simulink model "cooling_model"  (R2022a)
settings: Solver=VariableStepAuto  StartTime=4192  StopTime=20000  RelTol=1e-3
values from neighbouring files (symbols this model uses):
  area_air_fan = (fan_qty*pi.*fan_dia^2)./4'    [Cooling_Script.m]
  area_fins = n_fins * (h_fin-delta_fin) * w_radiator * 2    [Cooling_Script.m]
  area_fins_inverter = n_fins_inverter * (h_fin_inverter-delta_fin_inverter) * w_radiator_inverter * 2    [Cooling_Script.m]
  area_fins_motor = n_fins_motor * (h_fin_motor-delta_fin_motor) * w_radiator_motor * 2    [Cooling_Script.m]
  area_primary = 2 * L_tube * w_radiator * (n_fin_rows) - 2 * delta_fin * w_radiator * n_fins + 2 * h_fin * w_radiator * n_fin_rows + 2 * h_tube * n_tubes * L_tube    [Cooling_Script.m]
  area_primary_inverter = 2 * L_tube_inverter * w_radiator_inverter * (n_fin_rows_inverter) - 2 * delta_fin_inverter * w_radiator_inverter * n_fins_inverter + 2 * h_fin_inverter * w_radiator_inverter * n_fin_rows_inverter + 2 * h_tube_inverter * n_tubes_inverter * L_tube_inverter    [Cooling_Script.m]
  area_primary_motor = 2 * L_tube_motor * w_radiator_motor * (n_fin_rows_motor) - 2 * delta_fin_motor * w_radiator_motor * n_fins_motor + 2 * h_fin_motor * w_radiator_motor * n_fin_rows_motor + 2 * h_tube_motor * n_tubes_motor * L_tube_motor    [Cooling_Script.m]
  cp_air = 1004    [Cooling_Script.m]
  h_tube = 0.0015    [Cooling_Script.m]
  h_tube_inverter = 0.0015    [Cooling_Script.m]
  h_tube_motor = 0.0015    [Cooling_Script.m]
  HC_min = 10    [Cooling_Script.m]
  HC_nom = 100    [Cooling_Script.m]
  L_tube = 46*25.4./1000    [Cooling_Script.m]
  L_tube_inverter = 46*25.4./1000    [Cooling_Script.m]
  L_tube_motor = 46*25.4./1000    [Cooling_Script.m]
  n_tubes = 36    [Cooling_Script.m]
  n_tubes_inverter = 36    [Cooling_Script.m]
  n_tubes_motor = 36    [Cooling_Script.m]
  rho_air = 1.2    [Cooling_Script.m]
  vel_air_nom = 1    [Cooling_Script.m]
  w_radiator = 2.6*25.4    (= 66.04)    [Cooling_Script.m]
  w_radiator_inverter = 2.6*25.4    (= 66.04)    [Cooling_Script.m]
  w_radiator_motor = 2.6*25.4    (= 66.04)    [Cooling_Script.m]
libraries: fl_lib x65, nesl_utility x35, SimscapeFluids_lib x12, aerolibconvert2 x9
(part 2 of 2)

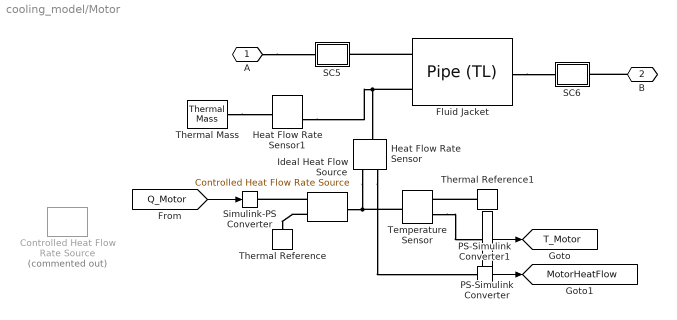
== system cooling_model/Motor ==
  Controlled Heat Flow Rate Source : fl_lib/Thermal/Thermal Sources/Controlled Heat Flow Rate Source  Commented=on
      settings: SourceProductBaseCode=PW,SS,VE
  Fluid Jacket : SimscapeFluids_lib/Thermal Liquid/Pipes & Fittings/Pipe (TL)  dynamic_compressibility=simscape.enum.onoff.off  inertia=simscape.enum.onoff.off  num_segments=1  pipe_length=0.2 m  area=pi*0.01^2 m^2  wall_spec=fluids.thermal_liquid.pipes_fittings.enum.wall_spec.rigid  Dh=0.005 m  wall_compliance=1.2e-6 m/MPa  wall_time_constant=0.01 s  elevation_spec=foundation.enum.constant_variable.constant  elevation_gain=0 m  g=9.81 m/s^2  pressure_loss_spec=fluids.thermal_liquid.pipes_fittings.enum.PressureLossSpec.Nominal  local_pressure_loss_spec=fluids.thermal_liquid.pipes_fittings.enum.LocalLossSpec.AggregateLength  length_add=0 m  loss_coefficient=0.1  roughness=1.5e-60 m  Re_friction_TLU=[ 400 1000 1.5e+3 3e+3 4e+3 6e+3 1e+4 2e+4 4e+4 6e+4 1e+5 1e+8 ]  friction_factor_TLU=[ 0.264 0.112 0.07099999999999999 0.0417 0.0387 0.0268 0.025 0.0232 0.0226 0.022 0.0214 0.0214 ]  shape_factor=1e-50  Re_lam=2e+3  Re_tur=4e+3  mdot_nominal=[ 0.1 1000 ] kg/s  p_diff_nominal=[ 0.00000001 0.000000001 ] MPa  mdot_threshold=1e-6 kg/s  heat_transfer_spec=fluids.thermal_liquid.pipes_fittings.enum.HeatTransferSpec.TabulatedNusselt  mdot_nominal_heat=[ 0.1 1 ] kg/s  T_in_nominal=[ 293.15 293.15 ] K  T_out_nominal=[ 300 300 ] K  p_in_nominal_heat=[ 0.101325 0.101325 ] MPa  T_wall_nominal=[ 303.15 303.15 ] K  a_coeff=0.023  b_Re_power=0.8  c_Pr_power=0.4  Nu_lam=3.66  Re_Colburn_TLU=[ 100 150 1000 ]  Colburn_factor_TLU=[ 0.019 0.013 0.002 ]  Re_Nu_TLU=Re_TLU  Pr_Nu_TLU=Pr_TLU  Nu_TLU=Nu_TLU  T0_vec=303.15 K  p0_vec=0.101325 MPa  mdot0=0.1 kg/s
      settings: SourceProductBaseCode=SH
  Heat Flow Rate Sensor : fl_lib/Thermal/Thermal Sensors/Heat Flow Rate Sensor
      settings: SourceProductBaseCode=PW,SS,VE
  Heat Flow Rate Sensor1 : fl_lib/Thermal/Thermal Sensors/Heat Flow Rate Sensor
      settings: SourceProductBaseCode=PW,SS,VE
  Ideal Heat Flow Source : fl_lib/Thermal/Thermal Sources/Controlled Heat Flow Rate Source
      settings: SourceProductBaseCode=PW,SS,VE
  PS-Simulink Converter : nesl_utility/PS-Simulink Converter  PhysicalDomain=network_engine_domain  SubClassName=ps_output  LeftPortType=input  RightPortType=output  PseudoPeriodic=off  Frequencies=[]  VectorFormat=1-D array  Unit=degC  AffineConversion=on
      settings: SourceProductBaseCode=SS,PW,VE
  PS-Simulink Converter1 : nesl_utility/PS-Simulink Converter  PhysicalDomain=network_engine_domain  SubClassName=ps_output  LeftPortType=input  RightPortType=output  PseudoPeriodic=off  Frequencies=[]  VectorFormat=inherit  Unit=inherit  AffineConversion=off
      settings: SourceProductBaseCode=SS,PW,VE
  SC5 : Subsystem
      mask Display: disp(get_param(gcb, 'Name'))
  SC6 : Subsystem
      mask Display: disp(get_param(gcb, 'Name'))
  Simulink-PS Converter : nesl_utility/Simulink-PS Converter  PhysicalDomain=network_engine_domain  SubClassName=ps_input  LeftPortType=input  RightPortType=output  PseudoPeriodic=off  Frequencies=[]  NoiseDistribution=none  NoiseParameters=[]  Unit=W  AffineConversion=off  FilteringAndDerivatives=provide  SimscapeFilterOrder=1  InputFilterTimeConstant=0.001  UdotUserProvided=0
      settings: SourceProductBaseCode=SS,PW,VE
  Temperature Sensor : fl_lib/Thermal/Thermal Sensors/Temperature Sensor
      settings: SourceProductBaseCode=PW,SS,VE
  Thermal Mass : fl_lib/Thermal/Thermal Elements/Thermal Mass  mass=28.5*6 kg  sp_heat=447 J/(K*kg)  T_specify=on  T_priority=High  T=273+45 K  T_nominal_specify=on  T_nominal_unit=K  T_nominal_value=273.15+45  Q_specify=off  Q_priority=None  Q=0 W  Q_nominal_specify=off  Q_nominal_unit=W  Q_nominal_value=1
      settings: SourceProductBaseCode=PW,SS,VE
  Thermal Reference : fl_lib/Thermal/Thermal Elements/Thermal Reference
      settings: SourceProductBaseCode=PW,SS,VE
  Thermal Reference1 : fl_lib/Thermal/Thermal Elements/Thermal Reference
      settings: SourceProductBaseCode=PW,SS,VE
  A : PMIOPort  Side=Left
  B : PMIOPort  Port=2  Side=Right
  tag scope: MotorHeatFlow=global, T_Motor=global
  wires:
  [Q_Motor] -> Simulink-PS Converter/1
  PS-Simulink Converter/1 -> [T_Motor]
  PS-Simulink Converter1/1 -> [MotorHeatFlow]
  connections:
  Temperature Sensor/LConn1 -- Heat Flow Rate Sensor/RConn2 -- Ideal Heat Flow Source/LConn1
  B/RConn1 -- SC6/RConn1
  Ideal Heat Flow Source/RConn2 -- Thermal Reference/LConn1
  A/RConn1 -- SC5/LConn1
  Ideal Heat Flow Source/RConn1 -- Simulink-PS Converter/RConn1
  Thermal Reference1/LConn1 -- Temperature Sensor/RConn1
  Temperature Sensor/RConn2 -- PS-Simulink Converter/LConn1
  Fluid Jacket/LConn2 -- Heat Flow Rate Sensor1/RConn2 -- Heat Flow Rate Sensor/LConn1
  Heat Flow Rate Sensor/RConn1 -- PS-Simulink Converter1/LConn1
  Fluid Jacket/LConn1 -- SC5/RConn1
  Fluid Jacket/RConn1 -- SC6/LConn1
  Thermal Mass/LConn1 -- Heat Flow Rate Sensor1/LConn1

== system cooling_model/Sensing Coolant1 ==
  Absolute Reference (TL) : fl_lib/Thermal Liquid/Elements/Absolute Reference (TL)
      settings: SourceProductBaseCode=PW,SS,VE
  PS-Simulink Converter : nesl_utility/PS-Simulink Converter  PhysicalDomain=network_engine_domain  SubClassName=ps_output  LeftPortType=input  RightPortType=output  PseudoPeriodic=off  Frequencies=[]  VectorFormat=1-D array  Unit=K  AffineConversion=on
      settings: SourceProductBaseCode=SS,PW,VE
  Pressure & Temperature Sensor (TL) : fl_lib/Thermal Liquid/Sensors/Pressure & Temperature Sensor (TL)
      settings: SourceProductBaseCode=PW,SS,VE  InternalSimscapePortConfiguration="{\"Bottom\":[],\"Left\":[{\"id\":\"A\",\"label\":\"A\",\"type\":\"foundation.thermal_liquid.thermal_liquid\"}],\"Right\":[{\"id\":\"B\",\"label\":\"B\",\"type\":\"foundation.thermal_liquid.thermal_liquid\"},{\"id\":\"P\",\"label\":\"P\",\"type\":\"output\"},{\"id\":\"T\",\"label\":\"T\",\"type\":\"output\"}],\"Top\":[]}"
  Conn1 : PMIOPort  Side=Left
  Out1 : Outport  VectorParamsAs1DForOutWhenUnconnected=off
  wires:
  PS-Simulink Converter/1 -> Out1/1
  connections:
  Pressure & Temperature Sensor (TL)/LConn1 -- Conn1/RConn1
  PS-Simulink Converter/LConn1 -- Pressure & Temperature Sensor (TL)/RConn3
  Pressure & Temperature Sensor (TL)/RConn1 -- Absolute Reference (TL)/LConn1

== system cooling_model/Sensing Coolant2 ==
  Absolute Reference (TL) : fl_lib/Thermal Liquid/Elements/Absolute Reference (TL)
      settings: SourceProductBaseCode=PW,SS,VE
  PS-Simulink Converter : nesl_utility/PS-Simulink Converter  PhysicalDomain=network_engine_domain  SubClassName=ps_output  LeftPortType=input  RightPortType=output  PseudoPeriodic=off  Frequencies=[]  VectorFormat=1-D array  Unit=K  AffineConversion=on
      settings: SourceProductBaseCode=SS,PW,VE
  Pressure & Temperature Sensor (TL) : fl_lib/Thermal Liquid/Sensors/Pressure & Temperature Sensor (TL)
      settings: SourceProductBaseCode=PW,SS,VE  InternalSimscapePortConfiguration="{\"Bottom\":[],\"Left\":[{\"id\":\"A\",\"label\":\"A\",\"type\":\"foundation.thermal_liquid.thermal_liquid\"}],\"Right\":[{\"id\":\"B\",\"label\":\"B\",\"type\":\"foundation.thermal_liquid.thermal_liquid\"},{\"id\":\"P\",\"label\":\"P\",\"type\":\"output\"},{\"id\":\"T\",\"label\":\"T\",\"type\":\"output\"}],\"Top\":[]}"
  Conn1 : PMIOPort  Side=Left
  Out1 : Outport  VectorParamsAs1DForOutWhenUnconnected=off
  wires:
  PS-Simulink Converter/1 -> Out1/1
  connections:
  Pressure & Temperature Sensor (TL)/LConn1 -- Conn1/RConn1
  PS-Simulink Converter/LConn1 -- Pressure & Temperature Sensor (TL)/RConn3
  Pressure & Temperature Sensor (TL)/RConn1 -- Absolute Reference (TL)/LConn1

== system cooling_model/Sensing Coolant3 ==
  Absolute Reference (TL) : fl_lib/Thermal Liquid/Elements/Absolute Reference (TL)
      settings: SourceProductBaseCode=PW,SS,VE
  PS-Simulink Converter : nesl_utility/PS-Simulink Converter  PhysicalDomain=network_engine_domain  SubClassName=ps_output  LeftPortType=input  RightPortType=output  PseudoPeriodic=off  Frequencies=[]  VectorFormat=1-D array  Unit=K  AffineConversion=on
      settings: SourceProductBaseCode=SS,PW,VE
  Pressure & Temperature Sensor (TL) : fl_lib/Thermal Liquid/Sensors/Pressure & Temperature Sensor (TL)
      settings: SourceProductBaseCode=PW,SS,VE  InternalSimscapePortConfiguration="{\"Bottom\":[],\"Left\":[{\"id\":\"A\",\"label\":\"A\",\"type\":\"foundation.thermal_liquid.thermal_liquid\"}],\"Right\":[{\"id\":\"B\",\"label\":\"B\",\"type\":\"foundation.thermal_liquid.thermal_liquid\"},{\"id\":\"P\",\"label\":\"P\",\"type\":\"output\"},{\"id\":\"T\",\"label\":\"T\",\"type\":\"output\"}],\"Top\":[]}"
  Conn1 : PMIOPort  Side=Left
  Out1 : Outport  VectorParamsAs1DForOutWhenUnconnected=off
  wires:
  PS-Simulink Converter/1 -> Out1/1
  connections:
  Pressure & Temperature Sensor (TL)/RConn1 -- Absolute Reference (TL)/LConn1
  PS-Simulink Converter/LConn1 -- Pressure & Temperature Sensor (TL)/RConn3
  Pressure & Temperature Sensor (TL)/LConn1 -- Conn1/RConn1

== system cooling_model/Engine1/SC5 ==
  Absolute Reference (TL) : fl_lib/Thermal Liquid/Elements/Absolute Reference (TL)
      settings: SourceProductBaseCode=PW,SS,VE
  Mass & Energy Flow Rate Sensor (TL) : fl_lib/Thermal Liquid/Sensors/Mass & Energy Flow Rate Sensor (TL)
      settings: SourceProductBaseCode=PW,SS,VE  InternalSimscapePortConfiguration="{\"Bottom\":[],\"Left\":[{\"id\":\"A\",\"label\":\"A\",\"type\":\"foundation.thermal_liquid.thermal_liquid\"}],\"Right\":[{\"id\":\"B\",\"label\":\"B\",\"type\":\"foundation.thermal_liquid.thermal_liquid\"},{\"id\":\"M\",\"label\":\"M\",\"type\":\"output\"},{\"id\":\"PHI\",\"label\":\"Phi\",\"type\":\"output\"}],\"Top\":[]}"
  PS-Simulink Converter : nesl_utility/PS-Simulink Converter  PhysicalDomain=network_engine_domain  SubClassName=ps_output  LeftPortType=input  RightPortType=output  PseudoPeriodic=off  Frequencies=[]  VectorFormat=1-D array  Unit=W  AffineConversion=off
      settings: SourceProductBaseCode=SS,PW,VE
  PS-Simulink Converter1 : nesl_utility/PS-Simulink Converter  PhysicalDomain=network_engine_domain  SubClassName=ps_output  LeftPortType=input  RightPortType=output  PseudoPeriodic=off  Frequencies=[]  VectorFormat=1-D array  Unit=K  AffineConversion=off
      settings: SourceProductBaseCode=SS,PW,VE
  Pressure & Temperature Sensor (TL) : fl_lib/Thermal Liquid/Sensors/Pressure & Temperature Sensor (TL)
      settings: SourceProductBaseCode=PW,SS,VE  InternalSimscapePortConfiguration="{\"Bottom\":[],\"Left\":[{\"id\":\"A\",\"label\":\"A\",\"type\":\"foundation.thermal_liquid.thermal_liquid\"}],\"Right\":[{\"id\":\"B\",\"label\":\"B\",\"type\":\"foundation.thermal_liquid.thermal_liquid\"},{\"id\":\"P\",\"label\":\"P\",\"type\":\"output\"},{\"id\":\"T\",\"label\":\"T\",\"type\":\"output\"}],\"Top\":[]}"
  A : PMIOPort  Side=Left
  B : PMIOPort  Port=2  Side=Right
  tag scope: Phi_motor_in=global, Temp_Engine_Coolant_Hose=global
  wires:
  PS-Simulink Converter/1 -> [Phi_motor_in]
  PS-Simulink Converter1/1 -> [Temp_Engine_Coolant_Hose]
  connections:
  Pressure & Temperature Sensor (TL)/LConn1 -- A/RConn1 -- Mass & Energy Flow Rate Sensor (TL)/LConn1
  Mass & Energy Flow Rate Sensor (TL)/RConn1 -- B/RConn1
  Absolute Reference (TL)/LConn1 -- Pressure & Temperature Sensor (TL)/RConn1
  Mass & Energy Flow Rate Sensor (TL)/RConn3 -- PS-Simulink Converter/LConn1
  PS-Simulink Converter1/LConn1 -- Pressure & Temperature Sensor (TL)/RConn3

== system cooling_model/Engine1/SC6 ==
  Absolute Reference (TL) : fl_lib/Thermal Liquid/Elements/Absolute Reference (TL)
      settings: SourceProductBaseCode=PW,SS,VE
  Mass & Energy Flow Rate Sensor (TL) : fl_lib/Thermal Liquid/Sensors/Mass & Energy Flow Rate Sensor (TL)
      settings: SourceProductBaseCode=PW,SS,VE  InternalSimscapePortConfiguration="{\"Bottom\":[],\"Left\":[{\"id\":\"A\",\"label\":\"A\",\"type\":\"foundation.thermal_liquid.thermal_liquid\"}],\"Right\":[{\"id\":\"B\",\"label\":\"B\",\"type\":\"foundation.thermal_liquid.thermal_liquid\"},{\"id\":\"M\",\"label\":\"M\",\"type\":\"output\"},{\"id\":\"PHI\",\"label\":\"Phi\",\"type\":\"output\"}],\"Top\":[]}"
  PS-Simulink Converter : nesl_utility/PS-Simulink Converter  PhysicalDomain=network_engine_domain  SubClassName=ps_output  LeftPortType=input  RightPortType=output  PseudoPeriodic=off  Frequencies=[]  VectorFormat=1-D array  Unit=W  AffineConversion=off
      settings: SourceProductBaseCode=SS,PW,VE
  PS-Simulink Converter2 : nesl_utility/PS-Simulink Converter  PhysicalDomain=network_engine_domain  SubClassName=ps_output  LeftPortType=input  RightPortType=output  PseudoPeriodic=off  Frequencies=[]  VectorFormat=1-D array  Unit=K  AffineConversion=off
      settings: SourceProductBaseCode=SS,PW,VE
  Pressure & Temperature Sensor (TL) : fl_lib/Thermal Liquid/Sensors/Pressure & Temperature Sensor (TL)
      settings: SourceProductBaseCode=PW,SS,VE  InternalSimscapePortConfiguration="{\"Bottom\":[],\"Left\":[{\"id\":\"A\",\"label\":\"A\",\"type\":\"foundation.thermal_liquid.thermal_liquid\"}],\"Right\":[{\"id\":\"B\",\"label\":\"B\",\"type\":\"foundation.thermal_liquid.thermal_liquid\"},{\"id\":\"P\",\"label\":\"P\",\"type\":\"output\"},{\"id\":\"T\",\"label\":\"T\",\"type\":\"output\"}],\"Top\":[]}"
  A : PMIOPort  Side=Left
  B : PMIOPort  Port=2  Side=Right
  tag scope: Phi_motor_out=global, Temp_Engine_Coolant_Out_Hose=global
  wires:
  PS-Simulink Converter/1 -> [Phi_motor_out]
  PS-Simulink Converter2/1 -> [Temp_Engine_Coolant_Out_Hose]
  connections:
  Pressure & Temperature Sensor (TL)/LConn1 -- A/RConn1 -- Mass & Energy Flow Rate Sensor (TL)/LConn1
  Mass & Energy Flow Rate Sensor (TL)/RConn1 -- B/RConn1
  Absolute Reference (TL)/LConn1 -- Pressure & Temperature Sensor (TL)/RConn1
  Mass & Energy Flow Rate Sensor (TL)/RConn3 -- PS-Simulink Converter/LConn1
  PS-Simulink Converter2/LConn1 -- Pressure & Temperature Sensor (TL)/RConn3

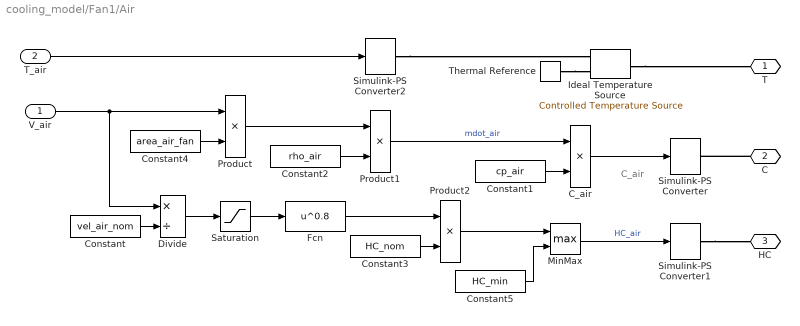
== system cooling_model/Fan1/Air ==
  note: C_air
  V_air : Inport
  T_air : Inport  Port=2
  C_air : Product
  Constant : Constant  Value=vel_air_nom
  Constant1 : Constant  Value=cp_air
  Constant2 : Constant  Value=rho_air
  Constant3 : Constant  Value=HC_nom
  Constant4 : Constant  Value=area_air_fan
  Constant5 : Constant  Value=HC_min
  Divide : Product  Inputs=*/
  Fcn : Fcn  Expr=u^0.8
  Ideal Temperature Source : fl_lib/Thermal/Thermal Sources/Controlled Temperature Source
      settings: SourceProductBaseCode=PW,SS,VE
  MinMax : MinMax  Function=max  Inputs=2
  Product : Product
  Product1 : Product
  Product2 : Product
  Saturation : Saturate  UpperLimit=inf  LowerLimit=0
  Simulink-PS Converter : nesl_utility/Simulink-PS Converter  PhysicalDomain=network_engine_domain  SubClassName=ps_input  LeftPortType=input  RightPortType=output  PseudoPeriodic=off  Frequencies=[]  NoiseDistribution=none  NoiseParameters=[]  Unit=W/K  AffineConversion=off  FilteringAndDerivatives=zero  SimscapeFilterOrder=1  InputFilterTimeConstant=1  UdotUserProvided=1
      settings: SourceProductBaseCode=SS,PW,VE
  Simulink-PS Converter1 : nesl_utility/Simulink-PS Converter  PhysicalDomain=network_engine_domain  SubClassName=ps_input  LeftPortType=input  RightPortType=output  PseudoPeriodic=off  Frequencies=[]  NoiseDistribution=none  NoiseParameters=[]  Unit=W/(m^2*K)  AffineConversion=off  FilteringAndDerivatives=zero  SimscapeFilterOrder=1  InputFilterTimeConstant=1  UdotUserProvided=1
      settings: SourceProductBaseCode=SS,PW,VE
  Simulink-PS Converter2 : nesl_utility/Simulink-PS Converter  PhysicalDomain=network_engine_domain  SubClassName=ps_input  LeftPortType=input  RightPortType=output  PseudoPeriodic=off  Frequencies=[]  NoiseDistribution=none  NoiseParameters=[]  Unit=K  AffineConversion=on  FilteringAndDerivatives=zero  SimscapeFilterOrder=1  InputFilterTimeConstant=1  UdotUserProvided=1
      settings: SourceProductBaseCode=SS,PW,VE
  Thermal Reference : fl_lib/Thermal/Thermal Elements/Thermal Reference
      settings: SourceProductBaseCode=PW,SS,VE
  T : PMIOPort  Side=Right
  C : PMIOPort  Port=2  Side=Right
  HC : PMIOPort  Port=3  Side=Right
  wires:
  Saturation/1 -> Fcn/1
  Product1/1 -> C_air/1  "mdot_air"
  Constant4/1 -> Product/2
  Constant2/1 -> Product1/2
  Product/1 -> Product1/1
  C_air/1 -> Simulink-PS Converter/1
  Constant1/1 -> C_air/2
  T_air/1 -> Simulink-PS Converter2/1
  MinMax/1 -> Simulink-PS Converter1/1  "HC_air"
  Constant5/1 -> MinMax/2
  Product2/1 -> MinMax/1
  Fcn/1 -> Product2/1
  Divide/1 -> Saturation/1
  Constant3/1 -> Product2/2
  Constant/1 -> Divide/2
  V_air/1 -> Divide/1, Product/1
  connections:
  Ideal Temperature Source/LConn1 -- T/RConn1
  Simulink-PS Converter2/RConn1 -- Ideal Temperature Source/RConn1
  Thermal Reference/LConn1 -- Ideal Temperature Source/RConn2
  Simulink-PS Converter1/RConn1 -- HC/RConn1
  C/RConn1 -- Simulink-PS Converter/RConn1

== system cooling_model/Fan1/Fan control ==
  V : Inport
  T : Inport  Port=2
  2-level fan controller : Subsystem
  A/C com : Constant  Value=0
  K : Constant  Value=273.15
  Subtract : Sum  Inputs=+-
  To Workspace : ToWorkspace  VariableName=Fan_volt  SampleTime=-1
  U_fan : Outport  VectorParamsAs1DForOutWhenUnconnected=off
  wires:
  2-level fan controller/1(U_fan) -> U_fan/1, To Workspace/1
  V/1 -> 2-level fan controller/1(V)
  Subtract/1 -> 2-level fan controller/2(T)
  A/C com/1 -> 2-level fan controller/3(A/C com)
  T/1 -> Subtract/1
  K/1 -> Subtract/2

== system cooling_model/Fan1/Fan unit ==
  note: Gain calculated by finding CFM of fan multipling by air density, then divide by default m_dot of air in the other block 0.246
  Veh_speed : Inport
  U_fan : Inport  Port=2
  2D Lookup Table : Lookup_n-D  LookupTableObject=''  BreakpointsForDimension1=[0,40,90,110,150,180,198]  BreakpointsForDimension2=[0 14.4]  Table=[0,0.8,2.2,2.7,3.6,4.1,4.6; 1.5,2.3,3.2,3.5,4.3,4.8,5.1]'  InternalRulePriority=Speed  RndMeth=Simplest
      settings: InputPortMap=u0,u1
  Gain : Gain  Gain=4
  Transfer Fcn : TransferFcn  Denominator=[10 1]
  V_air : Outport  VectorParamsAs1DForOutWhenUnconnected=off
  wires:
  Gain/1 -> V_air/1
  Transfer Fcn/1 -> Gain/1
  U_fan/1 -> 2D Lookup Table/2
  2D Lookup Table/1 -> Transfer Fcn/1
  Veh_speed/1 -> 2D Lookup Table/1

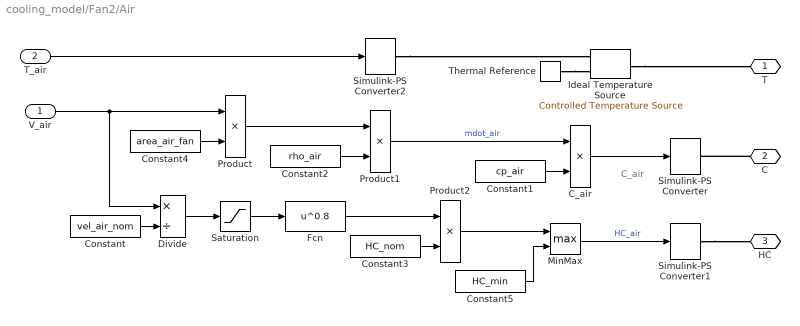
== system cooling_model/Fan2/Air ==
  note: C_air
  V_air : Inport
  T_air : Inport  Port=2
  C_air : Product
  Constant : Constant  Value=vel_air_nom
  Constant1 : Constant  Value=cp_air
  Constant2 : Constant  Value=rho_air
  Constant3 : Constant  Value=HC_nom
  Constant4 : Constant  Value=area_air_fan
  Constant5 : Constant  Value=HC_min
  Divide : Product  Inputs=*/
  Fcn : Fcn  Expr=u^0.8
  Ideal Temperature Source : fl_lib/Thermal/Thermal Sources/Controlled Temperature Source
      settings: SourceProductBaseCode=PW,SS,VE
  MinMax : MinMax  Function=max  Inputs=2
  Product : Product
  Product1 : Product
  Product2 : Product
  Saturation : Saturate  UpperLimit=inf  LowerLimit=0
  Simulink-PS Converter : nesl_utility/Simulink-PS Converter  PhysicalDomain=network_engine_domain  SubClassName=ps_input  LeftPortType=input  RightPortType=output  PseudoPeriodic=off  Frequencies=[]  NoiseDistribution=none  NoiseParameters=[]  Unit=W/K  AffineConversion=off  FilteringAndDerivatives=zero  SimscapeFilterOrder=1  InputFilterTimeConstant=1  UdotUserProvided=1
      settings: SourceProductBaseCode=SS,PW,VE
  Simulink-PS Converter1 : nesl_utility/Simulink-PS Converter  PhysicalDomain=network_engine_domain  SubClassName=ps_input  LeftPortType=input  RightPortType=output  PseudoPeriodic=off  Frequencies=[]  NoiseDistribution=none  NoiseParameters=[]  Unit=W/(m^2*K)  AffineConversion=off  FilteringAndDerivatives=zero  SimscapeFilterOrder=1  InputFilterTimeConstant=1  UdotUserProvided=1
      settings: SourceProductBaseCode=SS,PW,VE
  Simulink-PS Converter2 : nesl_utility/Simulink-PS Converter  PhysicalDomain=network_engine_domain  SubClassName=ps_input  LeftPortType=input  RightPortType=output  PseudoPeriodic=off  Frequencies=[]  NoiseDistribution=none  NoiseParameters=[]  Unit=K  AffineConversion=on  FilteringAndDerivatives=zero  SimscapeFilterOrder=1  InputFilterTimeConstant=1  UdotUserProvided=1
      settings: SourceProductBaseCode=SS,PW,VE
  Thermal Reference : fl_lib/Thermal/Thermal Elements/Thermal Reference
      settings: SourceProductBaseCode=PW,SS,VE
  T : PMIOPort  Side=Right
  C : PMIOPort  Port=2  Side=Right
  HC : PMIOPort  Port=3  Side=Right
  wires:
  V_air/1 -> Product/1, Divide/1
  Constant/1 -> Divide/2
  Constant3/1 -> Product2/2
  Divide/1 -> Saturation/1
  Fcn/1 -> Product2/1
  Product2/1 -> MinMax/1
  Constant5/1 -> MinMax/2
  MinMax/1 -> Simulink-PS Converter1/1  "HC_air"
  T_air/1 -> Simulink-PS Converter2/1
  Constant1/1 -> C_air/2
  C_air/1 -> Simulink-PS Converter/1
  Product/1 -> Product1/1
  Constant2/1 -> Product1/2
  Constant4/1 -> Product/2
  Product1/1 -> C_air/1  "mdot_air"
  Saturation/1 -> Fcn/1
  connections:
  C/RConn1 -- Simulink-PS Converter/RConn1
  Simulink-PS Converter1/RConn1 -- HC/RConn1
  Thermal Reference/LConn1 -- Ideal Temperature Source/RConn2
  Simulink-PS Converter2/RConn1 -- Ideal Temperature Source/RConn1
  Ideal Temperature Source/LConn1 -- T/RConn1

== system cooling_model/Fan2/Fan control ==
  V : Inport
  T : Inport  Port=2
  2-level fan controller : Subsystem
  A/C com : Constant  Value=0
  K : Constant  Value=273.15
  Subtract : Sum  Inputs=+-
  To Workspace : ToWorkspace  VariableName=Fan_volt  SampleTime=-1
  U_fan : Outport  VectorParamsAs1DForOutWhenUnconnected=off
  wires:
  K/1 -> Subtract/2
  T/1 -> Subtract/1
  A/C com/1 -> 2-level fan controller/3(A/C com)
  Subtract/1 -> 2-level fan controller/2(T)
  V/1 -> 2-level fan controller/1(V)
  2-level fan controller/1(U_fan) -> To Workspace/1, U_fan/1

== system cooling_model/Fan2/Fan unit ==
  note: Gain calculated by finding CFM of fan multipling by air density, then divide by default m_dot of air in the other block 0.246
  Veh_speed : Inport
  U_fan : Inport  Port=2
  2D Lookup Table : Lookup_n-D  LookupTableObject=''  BreakpointsForDimension1=[0,40,90,110,150,180,198]  BreakpointsForDimension2=[0 14.4]  Table=[0,0.8,2.2,2.7,3.6,4.1,4.6; 1.5,2.3,3.2,3.5,4.3,4.8,5.1]'  InternalRulePriority=Speed  RndMeth=Simplest
      settings: InputPortMap=u0,u1
  Gain : Gain  Gain=9.4
  Transfer Fcn : TransferFcn  Denominator=[10 1]
  V_air : Outport  VectorParamsAs1DForOutWhenUnconnected=off
  wires:
  Veh_speed/1 -> 2D Lookup Table/1
  2D Lookup Table/1 -> Transfer Fcn/1
  U_fan/1 -> 2D Lookup Table/2
  Transfer Fcn/1 -> Gain/1
  Gain/1 -> V_air/1

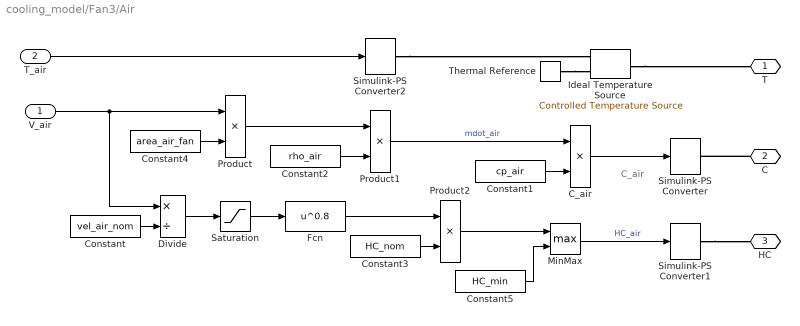
== system cooling_model/Fan3/Air ==
  note: C_air
  V_air : Inport
  T_air : Inport  Port=2
  C_air : Product
  Constant : Constant  Value=vel_air_nom
  Constant1 : Constant  Value=cp_air
  Constant2 : Constant  Value=rho_air
  Constant3 : Constant  Value=HC_nom
  Constant4 : Constant  Value=area_air_fan
  Constant5 : Constant  Value=HC_min
  Divide : Product  Inputs=*/
  Fcn : Fcn  Expr=u^0.8
  Ideal Temperature Source : fl_lib/Thermal/Thermal Sources/Controlled Temperature Source
      settings: SourceProductBaseCode=PW,SS,VE
  MinMax : MinMax  Function=max  Inputs=2
  Product : Product
  Product1 : Product
  Product2 : Product
  Saturation : Saturate  UpperLimit=inf  LowerLimit=0
  Simulink-PS Converter : nesl_utility/Simulink-PS Converter  PhysicalDomain=network_engine_domain  SubClassName=ps_input  LeftPortType=input  RightPortType=output  PseudoPeriodic=off  Frequencies=[]  NoiseDistribution=none  NoiseParameters=[]  Unit=W/K  AffineConversion=off  FilteringAndDerivatives=zero  SimscapeFilterOrder=1  InputFilterTimeConstant=1  UdotUserProvided=1
      settings: SourceProductBaseCode=SS,PW,VE
  Simulink-PS Converter1 : nesl_utility/Simulink-PS Converter  PhysicalDomain=network_engine_domain  SubClassName=ps_input  LeftPortType=input  RightPortType=output  PseudoPeriodic=off  Frequencies=[]  NoiseDistribution=none  NoiseParameters=[]  Unit=W/(m^2*K)  AffineConversion=off  FilteringAndDerivatives=zero  SimscapeFilterOrder=1  InputFilterTimeConstant=1  UdotUserProvided=1
      settings: SourceProductBaseCode=SS,PW,VE
  Simulink-PS Converter2 : nesl_utility/Simulink-PS Converter  PhysicalDomain=network_engine_domain  SubClassName=ps_input  LeftPortType=input  RightPortType=output  PseudoPeriodic=off  Frequencies=[]  NoiseDistribution=none  NoiseParameters=[]  Unit=K  AffineConversion=on  FilteringAndDerivatives=zero  SimscapeFilterOrder=1  InputFilterTimeConstant=1  UdotUserProvided=1
      settings: SourceProductBaseCode=SS,PW,VE
  Thermal Reference : fl_lib/Thermal/Thermal Elements/Thermal Reference
      settings: SourceProductBaseCode=PW,SS,VE
  T : PMIOPort  Side=Right
  C : PMIOPort  Port=2  Side=Right
  HC : PMIOPort  Port=3  Side=Right
  wires:
  Saturation/1 -> Fcn/1
  Product1/1 -> C_air/1  "mdot_air"
  Constant4/1 -> Product/2
  Constant2/1 -> Product1/2
  Product/1 -> Product1/1
  C_air/1 -> Simulink-PS Converter/1
  Constant1/1 -> C_air/2
  T_air/1 -> Simulink-PS Converter2/1
  MinMax/1 -> Simulink-PS Converter1/1  "HC_air"
  Constant5/1 -> MinMax/2
  Product2/1 -> MinMax/1
  Fcn/1 -> Product2/1
  Divide/1 -> Saturation/1
  Constant3/1 -> Product2/2
  Constant/1 -> Divide/2
  V_air/1 -> Divide/1, Product/1
  connections:
  Ideal Temperature Source/LConn1 -- T/RConn1
  Simulink-PS Converter2/RConn1 -- Ideal Temperature Source/RConn1
  Thermal Reference/LConn1 -- Ideal Temperature Source/RConn2
  Simulink-PS Converter1/RConn1 -- HC/RConn1
  C/RConn1 -- Simulink-PS Converter/RConn1

== system cooling_model/Fan3/Fan control ==
  V : Inport
  T : Inport  Port=2
  2-level fan controller : Subsystem
  A/C com : Constant  Value=0
  K : Constant  Value=273.15
  Subtract : Sum  Inputs=+-
  U_fan : Outport  VectorParamsAs1DForOutWhenUnconnected=off
  wires:
  2-level fan controller/1(U_fan) -> U_fan/1
  V/1 -> 2-level fan controller/1(V)
  Subtract/1 -> 2-level fan controller/2(T)
  A/C com/1 -> 2-level fan controller/3(A/C com)
  T/1 -> Subtract/1
  K/1 -> Subtract/2

== system cooling_model/Fan3/Fan unit ==
  note: Gain calculated by finding CFM of fan multipling by air density, then divide by default m_dot of air in the other block 0.246
  Veh_speed : Inport
  U_fan : Inport  Port=2
  2D Lookup Table : Lookup_n-D  LookupTableObject=''  BreakpointsForDimension1=[0,40,90,110,150,180,198]  BreakpointsForDimension2=[0 14.4]  Table=[0,0.8,2.2,2.7,3.6,4.1,4.6; 1.5,2.3,3.2,3.5,4.3,4.8,5.1]'  InternalRulePriority=Speed  RndMeth=Simplest
      settings: InputPortMap=u0,u1
  Gain : Gain  Gain=4
  Transfer Fcn : TransferFcn  Denominator=[10 1]
  V_air : Outport  VectorParamsAs1DForOutWhenUnconnected=off
  wires:
  Gain/1 -> V_air/1
  Transfer Fcn/1 -> Gain/1
  U_fan/1 -> 2D Lookup Table/2
  2D Lookup Table/1 -> Transfer Fcn/1
  Veh_speed/1 -> 2D Lookup Table/1

== system cooling_model/Inverter/SC5 ==
  Absolute Reference (TL) : fl_lib/Thermal Liquid/Elements/Absolute Reference (TL)
      settings: SourceProductBaseCode=PW,SS,VE
  Mass & Energy Flow Rate Sensor (TL) : fl_lib/Thermal Liquid/Sensors/Mass & Energy Flow Rate Sensor (TL)
      settings: SourceProductBaseCode=PW,SS,VE  InternalSimscapePortConfiguration="{\"Bottom\":[],\"Left\":[{\"id\":\"A\",\"label\":\"A\",\"type\":\"foundation.thermal_liquid.thermal_liquid\"}],\"Right\":[{\"id\":\"B\",\"label\":\"B\",\"type\":\"foundation.thermal_liquid.thermal_liquid\"},{\"id\":\"M\",\"label\":\"M\",\"type\":\"output\"},{\"id\":\"PHI\",\"label\":\"Phi\",\"type\":\"output\"}],\"Top\":[]}"
  PS-Simulink Converter1 : nesl_utility/PS-Simulink Converter  PhysicalDomain=network_engine_domain  SubClassName=ps_output  LeftPortType=input  RightPortType=output  PseudoPeriodic=off  Frequencies=[]  VectorFormat=1-D array  Unit=K  AffineConversion=off
      settings: SourceProductBaseCode=SS,PW,VE
  Pressure & Temperature Sensor (TL) : fl_lib/Thermal Liquid/Sensors/Pressure & Temperature Sensor (TL)
      settings: SourceProductBaseCode=PW,SS,VE  InternalSimscapePortConfiguration="{\"Bottom\":[],\"Left\":[{\"id\":\"A\",\"label\":\"A\",\"type\":\"foundation.thermal_liquid.thermal_liquid\"}],\"Right\":[{\"id\":\"B\",\"label\":\"B\",\"type\":\"foundation.thermal_liquid.thermal_liquid\"},{\"id\":\"P\",\"label\":\"P\",\"type\":\"output\"},{\"id\":\"T\",\"label\":\"T\",\"type\":\"output\"}],\"Top\":[]}"
  A : PMIOPort  Side=Left
  B : PMIOPort  Port=2  Side=Right
  tag scope: Inverter_Inlet=global
  wires:
  PS-Simulink Converter1/1 -> [Inverter_Inlet]
  connections:
  PS-Simulink Converter1/LConn1 -- Pressure & Temperature Sensor (TL)/RConn3
  Absolute Reference (TL)/LConn1 -- Pressure & Temperature Sensor (TL)/RConn1
  Mass & Energy Flow Rate Sensor (TL)/RConn1 -- B/RConn1
  Mass & Energy Flow Rate Sensor (TL)/LConn1 -- A/RConn1 -- Pressure & Temperature Sensor (TL)/LConn1

== system cooling_model/Inverter/SC6 ==
  Absolute Reference (TL) : fl_lib/Thermal Liquid/Elements/Absolute Reference (TL)
      settings: SourceProductBaseCode=PW,SS,VE
  Mass & Energy Flow Rate Sensor (TL) : fl_lib/Thermal Liquid/Sensors/Mass & Energy Flow Rate Sensor (TL)
      settings: SourceProductBaseCode=PW,SS,VE  InternalSimscapePortConfiguration="{\"Bottom\":[],\"Left\":[{\"id\":\"A\",\"label\":\"A\",\"type\":\"foundation.thermal_liquid.thermal_liquid\"}],\"Right\":[{\"id\":\"B\",\"label\":\"B\",\"type\":\"foundation.thermal_liquid.thermal_liquid\"},{\"id\":\"M\",\"label\":\"M\",\"type\":\"output\"},{\"id\":\"PHI\",\"label\":\"Phi\",\"type\":\"output\"}],\"Top\":[]}"
  PS-Simulink Converter2 : nesl_utility/PS-Simulink Converter  PhysicalDomain=network_engine_domain  SubClassName=ps_output  LeftPortType=input  RightPortType=output  PseudoPeriodic=off  Frequencies=[]  VectorFormat=1-D array  Unit=K  AffineConversion=off
      settings: SourceProductBaseCode=SS,PW,VE
  Pressure & Temperature Sensor (TL) : fl_lib/Thermal Liquid/Sensors/Pressure & Temperature Sensor (TL)
      settings: SourceProductBaseCode=PW,SS,VE  InternalSimscapePortConfiguration="{\"Bottom\":[],\"Left\":[{\"id\":\"A\",\"label\":\"A\",\"type\":\"foundation.thermal_liquid.thermal_liquid\"}],\"Right\":[{\"id\":\"B\",\"label\":\"B\",\"type\":\"foundation.thermal_liquid.thermal_liquid\"},{\"id\":\"P\",\"label\":\"P\",\"type\":\"output\"},{\"id\":\"T\",\"label\":\"T\",\"type\":\"output\"}],\"Top\":[]}"
  A : PMIOPort  Side=Left
  B : PMIOPort  Port=2  Side=Right
  tag scope: Inverter_Outlet=global
  wires:
  PS-Simulink Converter2/1 -> [Inverter_Outlet]
  connections:
  PS-Simulink Converter2/LConn1 -- Pressure & Temperature Sensor (TL)/RConn3
  Absolute Reference (TL)/LConn1 -- Pressure & Temperature Sensor (TL)/RConn1
  Mass & Energy Flow Rate Sensor (TL)/RConn1 -- B/RConn1
  Mass & Energy Flow Rate Sensor (TL)/LConn1 -- A/RConn1 -- Pressure & Temperature Sensor (TL)/LConn1

== system cooling_model/Motor/SC5 ==
  Absolute Reference (TL) : fl_lib/Thermal Liquid/Elements/Absolute Reference (TL)
      settings: SourceProductBaseCode=PW,SS,VE
  Mass & Energy Flow Rate Sensor (TL) : fl_lib/Thermal Liquid/Sensors/Mass & Energy Flow Rate Sensor (TL)
      settings: SourceProductBaseCode=PW,SS,VE  InternalSimscapePortConfiguration="{\"Bottom\":[],\"Left\":[{\"id\":\"A\",\"label\":\"A\",\"type\":\"foundation.thermal_liquid.thermal_liquid\"}],\"Right\":[{\"id\":\"B\",\"label\":\"B\",\"type\":\"foundation.thermal_liquid.thermal_liquid\"},{\"id\":\"M\",\"label\":\"M\",\"type\":\"output\"},{\"id\":\"PHI\",\"label\":\"Phi\",\"type\":\"output\"}],\"Top\":[]}"
  PS-Simulink Converter1 : nesl_utility/PS-Simulink Converter  PhysicalDomain=network_engine_domain  SubClassName=ps_output  LeftPortType=input  RightPortType=output  PseudoPeriodic=off  Frequencies=[]  VectorFormat=1-D array  Unit=K  AffineConversion=off
      settings: SourceProductBaseCode=SS,PW,VE
  Pressure & Temperature Sensor (TL) : fl_lib/Thermal Liquid/Sensors/Pressure & Temperature Sensor (TL)
      settings: SourceProductBaseCode=PW,SS,VE  InternalSimscapePortConfiguration="{\"Bottom\":[],\"Left\":[{\"id\":\"A\",\"label\":\"A\",\"type\":\"foundation.thermal_liquid.thermal_liquid\"}],\"Right\":[{\"id\":\"B\",\"label\":\"B\",\"type\":\"foundation.thermal_liquid.thermal_liquid\"},{\"id\":\"P\",\"label\":\"P\",\"type\":\"output\"},{\"id\":\"T\",\"label\":\"T\",\"type\":\"output\"}],\"Top\":[]}"
  A : PMIOPort  Side=Left
  B : PMIOPort  Port=2  Side=Right
  tag scope: T_Motor_Inlet=global
  wires:
  PS-Simulink Converter1/1 -> [T_Motor_Inlet]
  connections:
  Pressure & Temperature Sensor (TL)/LConn1 -- A/RConn1 -- Mass & Energy Flow Rate Sensor (TL)/LConn1
  Mass & Energy Flow Rate Sensor (TL)/RConn1 -- B/RConn1
  Absolute Reference (TL)/LConn1 -- Pressure & Temperature Sensor (TL)/RConn1
  PS-Simulink Converter1/LConn1 -- Pressure & Temperature Sensor (TL)/RConn3

== system cooling_model/Motor/SC6 ==
  Absolute Reference (TL) : fl_lib/Thermal Liquid/Elements/Absolute Reference (TL)
      settings: SourceProductBaseCode=PW,SS,VE
  Mass & Energy Flow Rate Sensor (TL) : fl_lib/Thermal Liquid/Sensors/Mass & Energy Flow Rate Sensor (TL)
      settings: SourceProductBaseCode=PW,SS,VE  InternalSimscapePortConfiguration="{\"Bottom\":[],\"Left\":[{\"id\":\"A\",\"label\":\"A\",\"type\":\"foundation.thermal_liquid.thermal_liquid\"}],\"Right\":[{\"id\":\"B\",\"label\":\"B\",\"type\":\"foundation.thermal_liquid.thermal_liquid\"},{\"id\":\"M\",\"label\":\"M\",\"type\":\"output\"},{\"id\":\"PHI\",\"label\":\"Phi\",\"type\":\"output\"}],\"Top\":[]}"
  PS-Simulink Converter2 : nesl_utility/PS-Simulink Converter  PhysicalDomain=network_engine_domain  SubClassName=ps_output  LeftPortType=input  RightPortType=output  PseudoPeriodic=off  Frequencies=[]  VectorFormat=1-D array  Unit=K  AffineConversion=off
      settings: SourceProductBaseCode=SS,PW,VE
  Pressure & Temperature Sensor (TL) : fl_lib/Thermal Liquid/Sensors/Pressure & Temperature Sensor (TL)
      settings: SourceProductBaseCode=PW,SS,VE  InternalSimscapePortConfiguration="{\"Bottom\":[],\"Left\":[{\"id\":\"A\",\"label\":\"A\",\"type\":\"foundation.thermal_liquid.thermal_liquid\"}],\"Right\":[{\"id\":\"B\",\"label\":\"B\",\"type\":\"foundation.thermal_liquid.thermal_liquid\"},{\"id\":\"P\",\"label\":\"P\",\"type\":\"output\"},{\"id\":\"T\",\"label\":\"T\",\"type\":\"output\"}],\"Top\":[]}"
  A : PMIOPort  Side=Left
  B : PMIOPort  Port=2  Side=Right
  tag scope: T_Motor_Outlet=global
  wires:
  PS-Simulink Converter2/1 -> [T_Motor_Outlet]
  connections:
  Pressure & Temperature Sensor (TL)/LConn1 -- A/RConn1 -- Mass & Energy Flow Rate Sensor (TL)/LConn1
  Mass & Energy Flow Rate Sensor (TL)/RConn1 -- B/RConn1
  Absolute Reference (TL)/LConn1 -- Pressure & Temperature Sensor (TL)/RConn1
  PS-Simulink Converter2/LConn1 -- Pressure & Temperature Sensor (TL)/RConn3

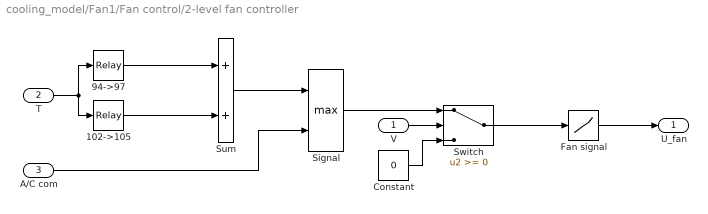
== system cooling_model/Fan1/Fan control/2-level fan controller ==
  V : Inport
  T : Inport  Port=2
  A/C com : Inport  Port=3
  102->105 : Relay  OnSwitchValue=20  OffSwitchValue=0
  94->97 : Relay  OnSwitchValue=20  OffSwitchValue=0
  Constant : Constant  Value=0
  Fan signal : Lookup  InputValues=[0, 1, 2]  Table=[0, 5, 14.4]
  Signal : MinMax  Function=max  Inputs=2  InputSameDT=on  SaturateOnIntegerOverflow=on
  Sum : Sum  Inputs=2  InputSameDT=on  SaturateOnIntegerOverflow=on  OutDataTypeStr=Inherit: Same as first input
  Switch : Switch  ZeroCross=off  SaturateOnIntegerOverflow=off  InputSameDT=off
  U_fan : Outport  VectorParamsAs1DForOutWhenUnconnected=off
  wires:
  Switch/1 -> Fan signal/1
  Constant/1 -> Switch/3
  V/1 -> Switch/2
  A/C com/1 -> Signal/2
  Signal/1 -> Switch/1
  Sum/1 -> Signal/1
  94->97/1 -> Sum/1
  102->105/1 -> Sum/2
  T/1 -> 94->97/1, 102->105/1
  Fan signal/1 -> U_fan/1

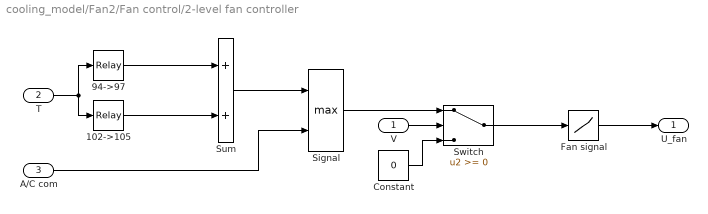
== system cooling_model/Fan2/Fan control/2-level fan controller ==
  V : Inport
  T : Inport  Port=2
  A/C com : Inport  Port=3
  102->105 : Relay  OnSwitchValue=90  OffSwitchValue=70
  94->97 : Relay  OnSwitchValue=80  OffSwitchValue=70
  Constant : Constant  Value=0
  Fan signal : Lookup  InputValues=[0, 1, 2]  Table=[0, 5, 14.4]
  Signal : MinMax  Function=max  Inputs=2  InputSameDT=on  SaturateOnIntegerOverflow=on
  Sum : Sum  Inputs=2  InputSameDT=on  SaturateOnIntegerOverflow=on  OutDataTypeStr=Inherit: Same as first input
  Switch : Switch  ZeroCross=off  SaturateOnIntegerOverflow=off  InputSameDT=off
  U_fan : Outport  VectorParamsAs1DForOutWhenUnconnected=off
  wires:
  Fan signal/1 -> U_fan/1
  T/1 -> 102->105/1, 94->97/1
  102->105/1 -> Sum/2
  94->97/1 -> Sum/1
  Sum/1 -> Signal/1
  Signal/1 -> Switch/1
  A/C com/1 -> Signal/2
  V/1 -> Switch/2
  Constant/1 -> Switch/3
  Switch/1 -> Fan signal/1

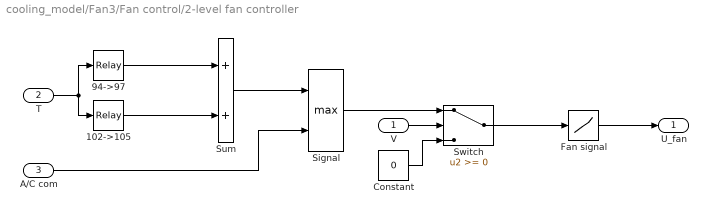
== system cooling_model/Fan3/Fan control/2-level fan controller ==
  V : Inport
  T : Inport  Port=2
  A/C com : Inport  Port=3
  102->105 : Relay  OnSwitchValue=20  OffSwitchValue=0
  94->97 : Relay  OnSwitchValue=20  OffSwitchValue=0
  Constant : Constant  Value=0
  Fan signal : Lookup  InputValues=[0, 1, 2]  Table=[0, 5, 14.4]
  Signal : MinMax  Function=max  Inputs=2  InputSameDT=on  SaturateOnIntegerOverflow=on
  Sum : Sum  Inputs=2  InputSameDT=on  SaturateOnIntegerOverflow=on  OutDataTypeStr=Inherit: Same as first input
  Switch : Switch  ZeroCross=off  SaturateOnIntegerOverflow=off  InputSameDT=off
  U_fan : Outport  VectorParamsAs1DForOutWhenUnconnected=off
  wires:
  Switch/1 -> Fan signal/1
  Constant/1 -> Switch/3
  V/1 -> Switch/2
  A/C com/1 -> Signal/2
  Signal/1 -> Switch/1
  Sum/1 -> Signal/1
  94->97/1 -> Sum/1
  102->105/1 -> Sum/2
  T/1 -> 94->97/1, 102->105/1
  Fan signal/1 -> U_fan/1
